simulink model "EnsayoControlVelocidad"  (R2022a)
settings: Solver=FixedStepAuto  StartTime=0.0  StopTime=inf  FixedStep=0.01  RelTol=1e-9  AbsTol=1e-9
PreLoadFcn:
  | setenv("RMW_IMPLEMENTATION","rmw_cyclonedds_cpp")
model workspace (MAT data in the model file):
  SL_ROS_VariableLengthArrays_MaxSizes.CommonInfo.ArrayTruncateAction = 'EmitWarning'
  SL_ROS_VariableLengthArrays_MaxSizes.MsgTypeMap = containers.Map
  SL_ROS_VariableLengthArrays_MaxSizes.MsgTypeMap.serialization.keys = {'sensor_msgs/LaserScan'}
  SL_ROS_VariableLengthArrays_MaxSizes.MsgTypeMap.serialization.values{1}(1).PropertyName = 'intensities'
  SL_ROS_VariableLengthArrays_MaxSizes.MsgTypeMap.serialization.values{1}(1).DataType = 'single'
  SL_ROS_VariableLengthArrays_MaxSizes.MsgTypeMap.serialization.values{1}(1).MaxLength = 360
  SL_ROS_VariableLengthArrays_MaxSizes.MsgTypeMap.serialization.values{1}(2).PropertyName = 'ranges'
  SL_ROS_VariableLengthArrays_MaxSizes.MsgTypeMap.serialization.values{1}(2).DataType = 'single'
  SL_ROS_VariableLengthArrays_MaxSizes.MsgTypeMap.serialization.values{1}(2).MaxLength = 360
  SL_ROS_VariableLengthArrays_MaxSizes.MsgTypeMap.serialization.uniformity = 0
  SL_ROS_VariableLengthArrays_MaxSizes.MsgTypeMap.serialization.keyType = 'char'
  SL_ROS_VariableLengthArrays_MaxSizes.MsgTypeMap.serialization.valueType = 'any'
values from neighbouring files (symbols this model uses):
  ref = 0.15    [plotEnsayosPC.m]
undefined symbols (not defined in the file or in its folder): header, twist
libraries: ros2lib x6
settings Model: Creator=Francisco  LastModifiedBy=Francisco
settings OptimizationCC: EnhancedBackFolding=on  PassReuseOutputArgsAs=Individual arguments  ZeroExternalMemoryAtStartup=off  ZeroInternalMemoryAtStartup=off  InitFltsAndDblsToZero=on  MaxStackSize=64  OptimizeBlockOrder=speed  DifferentSizesBufferReuse=on  OptimizationCustomize=off  EfficientTunableParamExpr=on
settings DebuggingCC: ParameterTunabilityLossMsg=error
settings HardwareCC: TargetLongLongMode=on
settings SFSimCC: MATLABDynamicMemAlloc=off
settings RTWCC: SystemTargetFile=ert.tlc  HardwareBoard=Robot Operating System 2 (ROS 2)  TLCOptions="-aInlineSetEventsForThisBaseRateFcn=TLC_FALSE -aSuppressMultiTaskScheduler=TLC_FALSE  -aRateBasedStepFcn=0"  TemplateMakefile=ert_default_tmf  GenerateReport=on  Toolchain=Colcon Tools  TargetLang=C++
settings CodeAppCC: ForceParamTrailComments=on  IgnoreCustomStorageClasses=off  OperatorAnnotations=on  SimulinkDataObjDesc=on  SFDataObjDesc=on  InsertBlockDesc=on
settings ERTTargetCC: CodeInterfacePackaging=C++ class  SupportContinuousTime=on  SupportNonInlinedSFcns=on  RootIOFormat=Structure reference

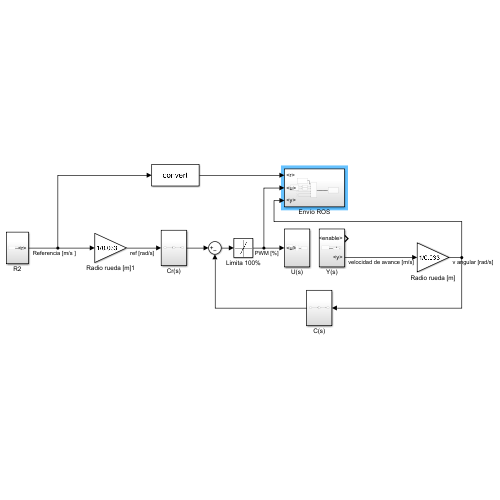
[thumbnail: Simulink's stored preview of the top-level diagram]
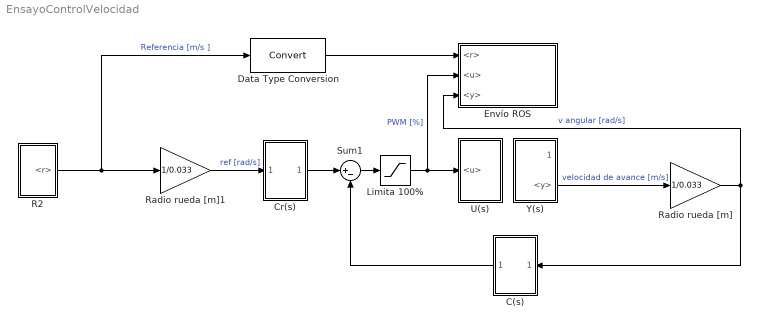
== system EnsayoControlVelocidad ==
  C(s) : Subsystem
  Cr(s) : Subsystem
  Data Type Conversion : DataTypeConversion  SaturateOnIntegerOverflow=off  RndMeth=Floor
  Envío ROS : Subsystem
  Limita 100% : Saturate  UpperLimit=100  LowerLimit=-100
  R2 : Subsystem
  Radio rueda [m] : Gain  Gain=1/0.033
  Radio rueda [m]1 : Gain  Gain=1/0.033  ParamDataTypeStr=double
  Sum1 : Sum  Inputs=|+-
  U(s) : Subsystem
  Y(s) : Subsystem
  wires:
  R2/1(<r>) -> Data Type Conversion/1, Radio rueda [m]1/1  "Referencia [m/s ]"
  Y(s)/2(<y>) -> Radio rueda [m]/1  "velocidad de avance [m/s]"
  Limita 100%/1 -> U(s)/1(<u>), Envío ROS/2(<u>)  "PWM [%]"
  Sum1/1 -> Limita 100%/1
  Radio rueda [m]/1 -> C(s)/1(" "), Envío ROS/3(<y>)  "v angular [rad/s]"
  Data Type Conversion/1 -> Envío ROS/1(<r>)
  C(s)/1("  ") -> Sum1/2
  Radio rueda [m]1/1 -> Cr(s)/1(" ")  "ref [rad/s]"
  Cr(s)/1("  ") -> Sum1/1

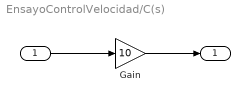
== system EnsayoControlVelocidad/C(s) ==
  " " : Inport
  Gain : Gain  Gain=10
  "  " : Outport
  wires:
  " "/1 -> Gain/1
  Gain/1 -> "  "/1

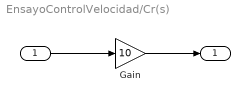
== system EnsayoControlVelocidad/Cr(s) ==
  " " : Inport
  Gain : Gain  Gain=10
  "  " : Outport
  wires:
  " "/1 -> Gain/1
  Gain/1 -> "  "/1

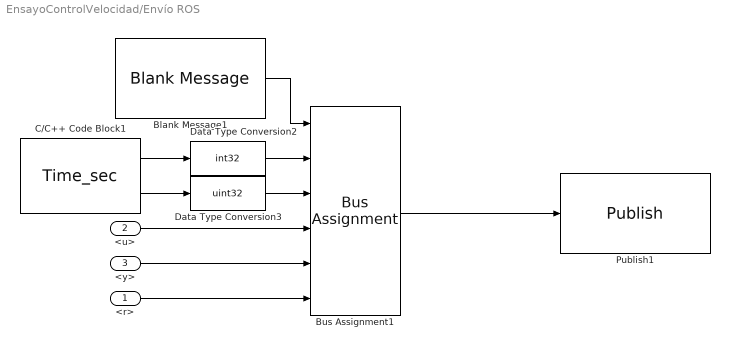
== system EnsayoControlVelocidad/Envío ROS ==
  <r> : Inport
  <u> : Inport  Port=2
  <y> : Inport  Port=3
  Blank Message1 : ros2lib/Blank Message  messageClass=Message  entityType=geometry_msgs/TwistStamped  messageType=geometry_msgs/TwistStamped  SampleTime=inf
      settings: SourceProductBaseCode=RR
  Bus Assignment1 : BusAssignment  AssignedSignals=header.stamp.sec,header.stamp.nanosec,twist.linear.x,twist.linear.y,twist.linear.z
  C/C++ Code Block1 : S-Function  FunctionName=Time_sec  SFunctionModules=Time_sec_wrapper  SFunctionDeploymentMode=off  EnableBusSupport=off  mask(S-Function Builder){}
      mask help: Simulink:masks:SFunctionBuilder_MD
      mask init:
      | val = [[.9  0.75 0.75 1 1 .9 .9 1]',[1 1 0.75 0.75 .9 .9 1 .9]'];try , sys = get_param(gcb,'SfunBuilderFcnName');if isempty(sys), sys = get_param(gcb,'FunctionName'); end,catch, sys = get_param(gcb,'FunctionName'); end
      settings: CopyFcn=set_param(gcbh,'LinkStatus','none')  OpenFcn=sfunctionwizard(gcbh)
      mask Display:
      | plot(val(:,1),val(:,2))
      | disp(sys)
      | port_label('output',1,'sec')
      | port_label('output',2,'nano')
  Data Type Conversion2 : DataTypeConversion  OutDataTypeStr=int32  SaturateOnIntegerOverflow=off  RndMeth=Floor
  Data Type Conversion3 : DataTypeConversion  OutDataTypeStr=uint32  SaturateOnIntegerOverflow=off  RndMeth=Floor
  Publish1 : ros2lib/Publish  topicSource=Specify your own  topic=/signals  messageType=geometry_msgs/TwistStamped  QOSHistory=Keep last  QOSDepth=1  QOSReliability=Reliable  QOSDurability=Volatile
      settings: SourceProductBaseCode=RR
  wires:
  <u>/1 -> Bus Assignment1/4
  Blank Message1/1 -> Bus Assignment1/1
  Bus Assignment1/1 -> Publish1/1
  Data Type Conversion2/1 -> Bus Assignment1/2
  C/C++ Code Block1/1 -> Data Type Conversion2/1
  Data Type Conversion3/1 -> Bus Assignment1/3
  C/C++ Code Block1/2 -> Data Type Conversion3/1
  <r>/1 -> Bus Assignment1/6
  <y>/1 -> Bus Assignment1/5

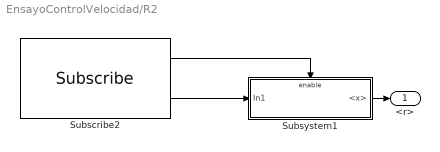
== system EnsayoControlVelocidad/R2 ==
  Subscribe2 : ros2lib/Subscribe  topicSource=Specify your own  topic=/ref  messageType=std_msgs/Float32  sampleTime=-1  QOSHistory=Keep last  QOSDepth=1  QOSReliability=Reliable  QOSDurability=Volatile
      settings: SourceProductBaseCode=RR
  Subsystem1 : Subsystem
  <r> : Outport
  wires:
  Subscribe2/1 -> Subsystem1/Enable
  Subscribe2/2 -> Subsystem1/1(In1)
  Subsystem1/1(<x>) -> <r>/1

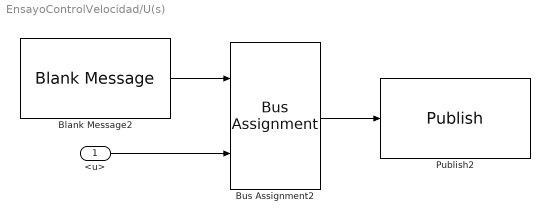
== system EnsayoControlVelocidad/U(s) ==
  <u> : Inport
  Blank Message2 : ros2lib/Blank Message  messageClass=Message  entityType=geometry_msgs/Twist  messageType=geometry_msgs/Twist  SampleTime=inf
      settings: SourceProductBaseCode=RR
  Bus Assignment2 : BusAssignment  AssignedSignals=linear.x
  Publish2 : ros2lib/Publish  topicSource=Select from ROS network  topic=/cmd_vel  messageType=geometry_msgs/Twist  QOSHistory=Keep last  QOSDepth=1  QOSReliability=Reliable  QOSDurability=Volatile
      settings: SourceProductBaseCode=RR
  wires:
  Bus Assignment2/1 -> Publish2/1
  Blank Message2/1 -> Bus Assignment2/1
  <u>/1 -> Bus Assignment2/2

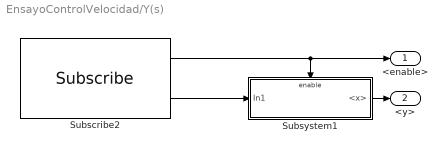
== system EnsayoControlVelocidad/Y(s) ==
  Subscribe2 : ros2lib/Subscribe  topicSource=Select from ROS network  topic=/joint_states  messageType=sensor_msgs/JointState  sampleTime=-1  QOSHistory=Keep last  QOSDepth=1  QOSReliability=Reliable  QOSDurability=Volatile
      settings: SourceProductBaseCode=RR
  Subsystem1 : Subsystem
  <enable> : Outport
  <y> : Outport  Port=2
  wires:
  Subscribe2/1 -> <enable>/1, Subsystem1/Enable
  Subscribe2/2 -> Subsystem1/1(In1)
  Subsystem1/1(<x>) -> <y>/1

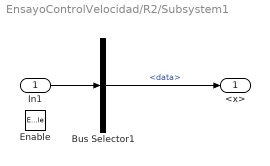
== system EnsayoControlVelocidad/R2/Subsystem1 ==
  In1 : Inport
  Enable : EnablePort
  Bus Selector1 : BusSelector  OutputSignals=data
  <x> : Outport
  wires:
  In1/1 -> Bus Selector1/1
  Bus Selector1/1 -> <x>/1  "<data>"

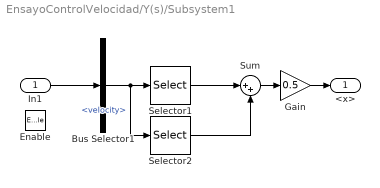
== system EnsayoControlVelocidad/Y(s)/Subsystem1 ==
  In1 : Inport
  Enable : EnablePort
  Bus Selector1 : BusSelector  OutputSignals=velocity
  Gain : Gain  Gain=0.5
  Selector1 : Selector  InputPortWidth=128  IndexOptions=Index vector (dialog)  Indices=[1]  OutputSizes=1  RuntimeRangeChecks=on
  Selector2 : Selector  InputPortWidth=128  IndexOptions=Index vector (dialog)  Indices=[2]  OutputSizes=1  RuntimeRangeChecks=on
  Sum : Sum  Inputs=|++
  <x> : Outport
  wires:
  In1/1 -> Bus Selector1/1
  Bus Selector1/1 -> Selector2/1, Selector1/1  "<velocity>"
  Selector1/1 -> Sum/1
  Selector2/1 -> Sum/2
  Sum/1 -> Gain/1
  Gain/1 -> <x>/1
